simulink model "Code_2DoF_Simulation_Discrete"  (R2016b)
settings: Solver=FixedStepDiscrete  StartTime=0  StopTime=32  FixedStep=0.0025  MaxStep=0.005  MinStep=0.001  RelTol=0.5
undefined symbols (not defined in the file or in its folder): DiscIntNeverNeededParam
settings Model: ExtModeTrigMode=oneshot  ExtModeArmWhenConnect=off  Creator=hp  LastModifiedBy=sfijdl
settings DataIOCC: ExternalInput=untitled.getElement(1),[],[],[],[],[],[],[],[],[],[],[],[],[],[],[],[],[],[]  SaveFormat=Array  SignalLoggingSaveFormat=ModelDataLogs  SignalLoggingName=sigsOut
settings OptimizationCC: DefaultParameterBehavior=Inlined  UseDivisionForNetSlopeComputation=on  UseFloatMulNetSlope=on  InlineInvariantSignals=on  PassReuseOutputArgsAs=Individual arguments  ExpressionDepthLimit=2147483647  ZeroExternalMemoryAtStartup=off  ZeroInternalMemoryAtStartup=off  NoFixptDivByZeroProtection=on  EfficientFloat2IntCast=on  LifeSpan=1
settings DebuggingCC: SaveWithParameterizedLinksMsg=none  UnderspecifiedInitializationDetection=Classic  MergeDetectMultiDrivingBlocksExec=none  SignalResolutionControl=TryResolveAllWithWarning  MultiTaskDSMMsg=warning  MultiTaskCondExecSysMsg=none  MultiTaskRateTransMsg=warning  ParameterTunabilityLossMsg=error  FcnCallInpInsideContextMsg=warning  StateNameClashWarn=warning  SFUnexpectedBacktrackingDiag=warning  SFNoUnconditionalDefaultTransitionDiag=warning  SFExecutionAtInitializationDiag=none
settings HardwareCC: TargetBitPerPointer=64  TargetBitPerSizeT=64  TargetBitPerPtrDiffT=64  TargetLongLongMode=on  TargetIntDivRoundTo=Zero  TargetEndianess=LittleEndian  TargetWordSize=64  TargetHWDeviceType=MATLAB Host  ProdEqTarget=off
settings ModelReferenceCC: PropagateSignalLabelsOutOfModel=off
settings RTWCC: SystemTargetFile=ert.tlc  TemplateMakefile=ert_default_tmf  Description=Embedded Coder  GenerateReport=on  IncludeHyperlinkInReport=on  LaunchReport=on  GenerateTraceInfo=on  GenerateTraceReport=on  GenerateTraceReportSl=on  GenerateTraceReportSf=on  GenerateTraceReportEml=on  GenerateCodeMetricsReport=on
settings CodeAppCC: ForceParamTrailComments=on  IgnoreCustomStorageClasses=off  MaxIdLength=128  OperatorAnnotations=on  SimulinkDataObjDesc=on  SFDataObjDesc=on  MATLABFcnDesc=on  CustomSymbolStrGlobalVar=rt$N$M  CustomSymbolStrType=$N$M  CustomSymbolStrFcn=$N$M$F  CustomSymbolStrMacro=$N$M  InsertBlockDesc=on  MATLABSourceComments=on
settings ERTTargetCC: GenerateSampleERTMain=on  CombineSignalStateStructs=on  SupportComplex=off  SupportNonInlinedSFcns=on  InlinedParameterPlacement=NonHierarchical  ERTCustomFileTemplate=example_file_process.tlc  ERTFilePackagingFormat=CompactWithDataFile
settings ConfigComp: CovMetricSettings=dw  CovHtmlReporting=on  CovSaveCumulativeToWorkspaceVar=on  CovSaveSingleToWorkspaceVar=on  CovExternalEMLEnable=off

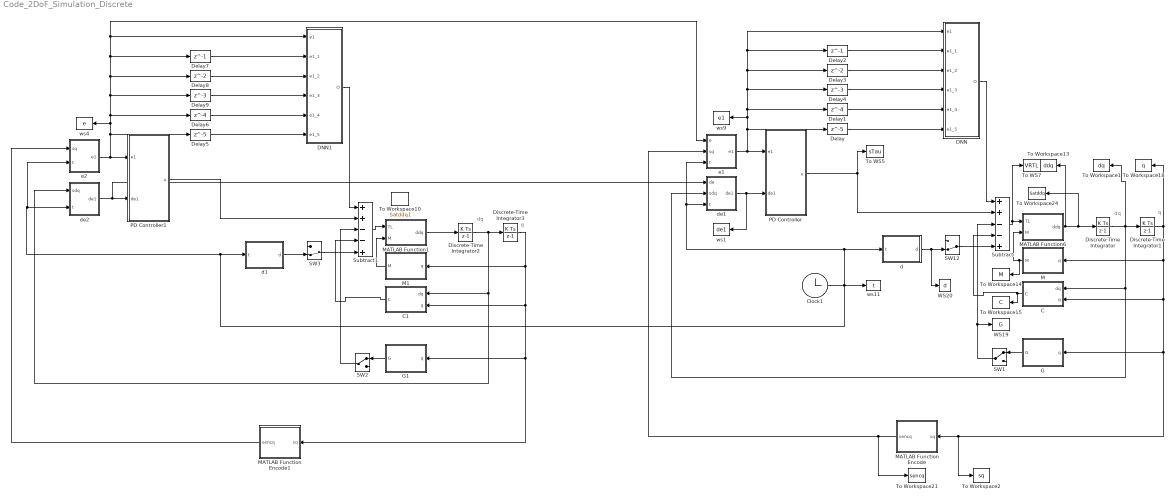
== system Code_2DoF_Simulation_Discrete ==
  note: q
  note: dq
  note: q
  note: dq
  C : MATLAB Function  TreatAsAtomicUnit=on
  C1 : MATLAB Function  TreatAsAtomicUnit=on
  Clock1 : Clock
  DNN : MATLAB Function  TreatAsAtomicUnit=on
  DNN1 : MATLAB Function  TreatAsAtomicUnit=on
  Delay : Delay  DelayLength=5  InitialCondition=0
  Delay1 : Delay  DelayLength=4  InitialCondition=0
  Delay2 : Delay  DelayLength=1  InitialCondition=0
  Delay3 : Delay  InitialCondition=0
  Delay4 : Delay  DelayLength=3  InitialCondition=0
  Delay5 : Delay  DelayLength=5  InitialCondition=0
  Delay6 : Delay  DelayLength=4  InitialCondition=0
  Delay7 : Delay  DelayLength=1  InitialCondition=0
  Delay8 : Delay  InitialCondition=0
  Delay9 : Delay  DelayLength=3  InitialCondition=0
  Discrete-Time Integrator : DiscreteIntegrator  InitialCondition=[0;0]  InitialConditionSetting=State (most efficient)  SampleTime=-1  ICPrevOutput=DiscIntNeverNeededParam  ICPrevScaledInput=DiscIntNeverNeededParam
  Discrete-Time Integrator1 : DiscreteIntegrator  InitialCondition=[-1;0]  InitialConditionSetting=State (most efficient)  SampleTime=-1  ICPrevOutput=DiscIntNeverNeededParam  ICPrevScaledInput=DiscIntNeverNeededParam
  Discrete-Time Integrator2 : DiscreteIntegrator  InitialCondition=[0;0]  InitialConditionSetting=State (most efficient)  SampleTime=-1  ICPrevOutput=DiscIntNeverNeededParam  ICPrevScaledInput=DiscIntNeverNeededParam
  Discrete-Time Integrator3 : DiscreteIntegrator  InitialCondition=[-1;0]  InitialConditionSetting=State (most efficient)  SampleTime=-1  ICPrevOutput=DiscIntNeverNeededParam  ICPrevScaledInput=DiscIntNeverNeededParam
  G : MATLAB Function  TreatAsAtomicUnit=on
  G1 : MATLAB Function  TreatAsAtomicUnit=on
  M : MATLAB Function  TreatAsAtomicUnit=on
  M1 : MATLAB Function  TreatAsAtomicUnit=on
  MATLAB Function Encode : MATLAB Function  TreatAsAtomicUnit=on
  MATLAB Function Encode1 : MATLAB Function  TreatAsAtomicUnit=on
  MATLAB Function1 : MATLAB Function  TreatAsAtomicUnit=on
  MATLAB Function6 : MATLAB Function  TreatAsAtomicUnit=on
  PD Controller : MATLAB Function  TreatAsAtomicUnit=on
  PD Controller1 : MATLAB Function  TreatAsAtomicUnit=on
  SW1 : ManualSwitch
  SW12 : ManualSwitch  CurrentSetting=0
  SW2 : ManualSwitch
  SW3 : ManualSwitch  CurrentSetting=0
  Subtract : Sum  Inputs=++--+
  Subtract1 : Sum  Inputs=++--+
  To WS5 : ToWorkspace  VariableName=sTau  SampleTime=-1
  To WS7 : ToWorkspace  VariableName=VRTL  SampleTime=-1
  To Workspace1 : ToWorkspace  VariableName=dq  SampleTime=-1
  To Workspace10 : ToWorkspace  VariableName=Satddq1  SampleTime=-1
  To Workspace13 : ToWorkspace  VariableName=ddq  SampleTime=-1
  To Workspace14 : ToWorkspace  VariableName=M  SampleTime=-1
  To Workspace15 : ToWorkspace  VariableName=C  SampleTime=-1
  To Workspace18 : ToWorkspace  VariableName=q  SampleTime=-1
  To Workspace2 : ToWorkspace  VariableName=sq  SampleTime=-1
  To Workspace21 : ToWorkspace  VariableName=sencq  SampleTime=-1
  To Workspace24 : ToWorkspace  VariableName=Satddq  SampleTime=-1
  WS19 : ToWorkspace  VariableName=G  SampleTime=-1
  WS20 : ToWorkspace  VariableName=d  SampleTime=-1
  d : MATLAB Function  TreatAsAtomicUnit=on
  d1 : MATLAB Function  TreatAsAtomicUnit=on
  de1 : MATLAB Function  TreatAsAtomicUnit=on
  de2 : MATLAB Function  TreatAsAtomicUnit=on
  e1 : MATLAB Function  TreatAsAtomicUnit=on
  e2 : MATLAB Function  TreatAsAtomicUnit=on
  ws1 : ToWorkspace  VariableName=de1  SampleTime=-1
  ws11 : ToWorkspace  VariableName=t  SampleTime=-1
  ws4 : ToWorkspace  VariableName=e  SampleTime=-1
  ws9 : ToWorkspace  VariableName=e1  SampleTime=-1
  wires:
  SW1/1 -> Subtract/3, WS19/1
  C/1(C) -> Subtract/4, To Workspace15/1
  Subtract/1 -> To WS7/1, MATLAB Function6/1(TL)
  M/1(M) -> MATLAB Function6/2(M), To Workspace14/1
  PD Controller/1(u) -> Subtract/2, To WS5/1
  Clock1/1 -> e2/2(t), de2/2(t), d1/1(t), ws11/1, e1/3(t), de1/3(t), d/1(t)
  Discrete-Time Integrator1/1 -> MATLAB Function Encode/1(sq), To Workspace2/1, G/1(q), C/2(q), M/1(q), To Workspace18/1
  MATLAB Function6/1(ddq) -> Discrete-Time Integrator/1, To Workspace24/1, To Workspace13/1
  de1/1(de1) -> ws1/1, PD Controller/2(de1)
  Discrete-Time Integrator/1 -> Discrete-Time Integrator1/1, To Workspace1/1, de1/2(sdq), C/1(dq)
  MATLAB Function Encode/1(sencq) -> To Workspace21/1, e1/2(sq)
  d/1(d) -> WS20/1, SW12/2
  SW12/1 -> Subtract/5
  G/1(G) -> SW1/1
  DNN/1(O) -> Subtract/1
  Delay/1 -> DNN/6(e1_5)
  Delay1/1 -> DNN/5(e1_4)
  Delay4/1 -> DNN/4(e1_3)
  Delay3/1 -> DNN/3(e1_2)
  Delay2/1 -> DNN/2(e1_1)
  e1/1(e1) -> PD Controller/1(e1), DNN/1(e1), Delay2/1, Delay3/1, Delay4/1, Delay1/1, ws9/1, Delay/1
  SW2/1 -> Subtract1/3
  C1/1(C) -> Subtract1/4
  Subtract1/1 -> MATLAB Function1/1(TL)
  M1/1(M) -> MATLAB Function1/2(M)
  PD Controller1/1(u) -> Subtract1/2
  Discrete-Time Integrator3/1 -> MATLAB Function Encode1/1(sq), G1/1(q), C1/2(q), M1/1(q)
  MATLAB Function1/1(ddq) -> Discrete-Time Integrator2/1
  de2/1(de1) -> de1/1(de), PD Controller1/2(de1)
  Discrete-Time Integrator2/1 -> Discrete-Time Integrator3/1, de2/1(sdq), C1/1(dq)
  MATLAB Function Encode1/1(sencq) -> e2/1(sq)
  d1/1(d) -> SW3/2
  SW3/1 -> Subtract1/5
  G1/1(G) -> SW2/1
  DNN1/1(O) -> Subtract1/1
  Delay5/1 -> DNN1/6(e1_5)
  Delay6/1 -> DNN1/5(e1_4)
  Delay9/1 -> DNN1/4(e1_3)
  Delay8/1 -> DNN1/3(e1_2)
  Delay7/1 -> DNN1/2(e1_1)
  e2/1(e1) -> PD Controller1/1(e1), e1/1(e), DNN1/1(e1), Delay7/1, Delay8/1, Delay9/1, Delay6/1, ws4/1, Delay5/1

== matlab function Code_2DoF_Simulation_Discrete/DNN ==
  settings: updateMethod=DISCRETE  sampleTime=0.0025
  data: e1 input; e1_1 input; e1_2 input; O output; e1_3 input; e1_4 input; e1_5 input
function O = DNN(e1,e1_1,e1_2,e1_3,e1_4,e1_5)
O=0;
end

== matlab function Code_2DoF_Simulation_Discrete/C1 ==
  settings: updateMethod=DISCRETE  sampleTime=0.0025
  data: dq input; C output; q input
function C = Col(dq,q)
q1=q(1);q2=q(2);
dq1=dq(1);dq2=dq(2);
s1=sin(q1);s2=sin(q2);
c1=cos(q1);c2=cos(q2);
m1=5;m2=5;
l1=1;l2=1;
g=9.81;
C11=-m2*l1*l2*s2*dq2;
C12=-m2*l1*l2*s2*dq2/2;
C21=m2*l1*l2*s2*dq1/2;
C22=0;
CM=[C11 C12
    C21 C22];
C=CM*dq;
end

== matlab function Code_2DoF_Simulation_Discrete/DNN1 ==
  settings: updateMethod=DISCRETE  sampleTime=0.0025
  data: e1 input; e1_1 input; e1_2 input; O output; e1_3 input; e1_4 input; e1_5 input
function O = DNN(e1,e1_1,e1_2,e1_3,e1_4,e1_5)
O=0;
end

== matlab function Code_2DoF_Simulation_Discrete/G1 ==
  settings: updateMethod=DISCRETE  sampleTime=0.0025
  data: q input; G output
function G = Gravity(q)
q1=q(1);q2=q(2);
s1=sin(q1);s2=sin(q2);
c1=cos(q1);c2=cos(q2);
c12=cos(q1+q2);
m1=5;m2=5;
l1=1;l2=1;
g=9.81;
G1 = m1*g*l1*c1/2+m2*g*l1*c1+m2*g*l2*c12/2; 
G2 = m2*g*l2*c12/2;
G=[G1;
   G2]; 
end

== matlab function Code_2DoF_Simulation_Discrete/M1 ==
  settings: updateMethod=DISCRETE  sampleTime=0.0025
  data: q input; M output
function M = Stiffness(q)
q1=q(1);q2=q(2);
s1=sin(q1);s2=sin(q2);
c1=cos(q1);c2=cos(q2);
m1=5;m2=5;
l1=1;l2=1;
g=9.81;
M11=m1*l1^2/3+m2*l1^2+m2*l2^2/4+m2*l1*l2*c2;
M12=m2*l2^2/4+m2*l1*l2*c2/2;
M22=m2*l2^2/3;
M = [M11; M12; 
     M12; M22];
end

== matlab function Code_2DoF_Simulation_Discrete/MATLAB Function Encode1 ==
  settings: updateMethod=DISCRETE  sampleTime=0.0025
  data: sq input; sencq output
function sencq = Enc(sq)
Delta=2*pi/2^19;
sencq=[0;0];
for i=1:1:2
    Number=floor(sq(i)/Delta)+1;
    sencq(i)=Number*Delta;
end
sencq=[sencq(1);sencq(2)];
% sencq=[sq(1);sq(2)];
end

== matlab function Code_2DoF_Simulation_Discrete/G ==
  settings: updateMethod=DISCRETE  sampleTime=0.0025
  data: q input; G output
function G = Gravity(q)
q1=q(1);q2=q(2);
s1=sin(q1);s2=sin(q2);
c1=cos(q1);c2=cos(q2);
c12=cos(q1+q2);
m1=5;m2=5;
l1=1;l2=1;
g=9.81;
G1 = m1*g*l1*c1/2+m2*g*l1*c1+m2*g*l2*c12/2; 
G2 = m2*g*l2*c12/2;
G=[G1;
   G2]; 
end

== matlab function Code_2DoF_Simulation_Discrete/MATLAB Function1 ==
  settings: updateMethod=DISCRETE  sampleTime=0.0025
  data: TL input; M input; ddq output
function ddq = Dynamics(TL,M)

M22 = [M(1) M(2)
       M(3) M(4)];
ddq=M22 \ TL;
end

== matlab function Code_2DoF_Simulation_Discrete/PD Controller1 ==
  settings: updateMethod=DISCRETE  sampleTime=0.0025
  data: e1 input; de1 input; u output
function u = Ctller(e1,de1)
% kp1=5000; kp2=1000; kd1=1000; kd2=80;
kp1=1000; kp2=800; kd1=500; kd2=80;
Kp=diag([kp1;kp2]);Kd=diag([kd1;kd2]);
u=-Kp*e1-Kd*de1;
end

== matlab function Code_2DoF_Simulation_Discrete/C ==
  settings: updateMethod=DISCRETE  sampleTime=0.0025
  data: dq input; C output; q input
function C = Col(dq,q)
q1=q(1);q2=q(2);
dq1=dq(1);dq2=dq(2);
s1=sin(q1);s2=sin(q2);
c1=cos(q1);c2=cos(q2);
m1=5;m2=5;
l1=1;l2=1;
g=9.81;
C11=-m2*l1*l2*s2*dq2;
C12=-m2*l1*l2*s2*dq2/2;
C21=m2*l1*l2*s2*dq1/2;
C22=0;
CM=[C11 C12
    C21 C22];
C=CM*dq;
end

== matlab function Code_2DoF_Simulation_Discrete/e1 ==
  settings: updateMethod=DISCRETE  sampleTime=0.0025
  data: e input; sq input; e1 output; t input
function e1 = e1(e,sq,t)
q=[sq(1);sq(2)];
qd1=sin(pi/4*t)-pi/2;
qd2=pi/2*cos(pi/8*(t+pi/2))*sin(pi/4*(t+pi/2));
% qd1=1;
% qd2=1;
qd=[qd1;qd2]; 
e1=q-qd;
e1=q-(qd-e1);
% e1=q-(qd-e);
end

== matlab function Code_2DoF_Simulation_Discrete/d1 ==
  settings: updateMethod=CONTINUOUS  sampleTime=0.0005
  data: t input; d output
function d = disturbance(t)
if t>10
% d=0.1*rand(6,1);
d=50.0*[sin(0.6*(t-10));sin(0.6*(t-10))];
else
    d=zeros(2,1);
% d=0.1*rand(6,1)*3*sin(0.5*t);
% d=0.3*sin(0.5*t)*ones(6,1);
end
end

== matlab function Code_2DoF_Simulation_Discrete/de2 ==
  settings: updateMethod=DISCRETE  sampleTime=0.0025
  data: sdq input; t input; de1 output
function de1 = de1(sdq,t)
dqd1=pi/4*cos(pi/4*t);
dqd2=pi/2*sin(pi/4*(t+pi/2))*-pi/8*sin(pi/8*(t+pi/2))+pi/2*cos(pi/8*(t+pi/2))*pi/4*cos(pi/4*(t+pi/2));
% dqd1=0;
% dqd2=0;
dqd=[dqd1;dqd2];
de1=sdq-dqd;
% de1=sdq-(dqd-de1);
end

== matlab function Code_2DoF_Simulation_Discrete/MATLAB Function6 ==
  settings: updateMethod=DISCRETE  sampleTime=0.0025
  data: TL input; M input; ddq output
function ddq = Dynamics(TL,M)

M22 = [M(1) M(2)
       M(3) M(4)];
ddq=M22 \ TL;
end

== matlab function Code_2DoF_Simulation_Discrete/e2 ==
  settings: updateMethod=DISCRETE  sampleTime=0.0025
  data: sq input; e1 output; t input
function e1 = e1(sq,t)
q=[sq(1);sq(2)];
qd1=sin(pi/4*t)-pi/2;
qd2=pi/2*cos(pi/8*(t+pi/2))*sin(pi/4*(t+pi/2));
% qd1=1;
% qd2=1;
qd=[qd1;qd2]; 
e1=q-qd;
% e1=q-(qd-e1);
end

== matlab function Code_2DoF_Simulation_Discrete/M ==
  settings: updateMethod=DISCRETE  sampleTime=0.0025
  data: q input; M output
function M = Stiffness(q)
q1=q(1);q2=q(2);
s1=sin(q1);s2=sin(q2);
c1=cos(q1);c2=cos(q2);
m1=5;m2=5;
l1=1;l2=1;
g=9.81;
M11=m1*l1^2/3+m2*l1^2+m2*l2^2/4+m2*l1*l2*c2;
M12=m2*l2^2/4+m2*l1*l2*c2/2;
M22=m2*l2^2/3;
M = [M11; M12; 
     M12; M22];
end

== matlab function Code_2DoF_Simulation_Discrete/d ==
  settings: updateMethod=CONTINUOUS  sampleTime=0.0005
  data: t input; d output
function d = disturbance(t)
if t>10
% d=0.1*rand(6,1);
d=50.0*[sin(0.6*(t-10));sin(0.6*(t-10))];
else
    d=zeros(2,1);
% d=0.1*rand(6,1)*3*sin(0.5*t);
% d=0.3*sin(0.5*t)*ones(6,1);
end
end

== matlab function Code_2DoF_Simulation_Discrete/MATLAB Function Encode ==
  settings: updateMethod=DISCRETE  sampleTime=0.0025
  data: sq input; sencq output
function sencq = Enc(sq)
Delta=2*pi/2^19;
sencq=[0;0];
for i=1:1:2
    Number=floor(sq(i)/Delta)+1;
    sencq(i)=Number*Delta;
end
sencq=[sencq(1);sencq(2)];
% sencq=[sq(1);sq(2)];
end

== matlab function Code_2DoF_Simulation_Discrete/PD Controller ==
  settings: updateMethod=DISCRETE  sampleTime=0.0025
  data: e1 input; de1 input; u output
function u = Ctller(e1,de1)
% kp1=5000; kp2=1000; kd1=1000; kd2=80;
kp1=1000; kp2=800; kd1=500; kd2=80;
Kp=diag([kp1;kp2]);Kd=diag([kd1;kd2]);
u=-Kp*e1-Kd*de1;
end

== matlab function Code_2DoF_Simulation_Discrete/de1 ==
  settings: updateMethod=DISCRETE  sampleTime=0.0025
  data: de input; sdq input; t input; de1 output
function de1 = de1(de,sdq,t)
dqd1=pi/4*cos(pi/4*t);
dqd2=pi/2*sin(pi/4*(t+pi/2))*-pi/8*sin(pi/8*(t+pi/2))+pi/2*cos(pi/8*(t+pi/2))*pi/4*cos(pi/4*(t+pi/2));
% dqd1=0;
% dqd2=0;
dqd=[dqd1;dqd2];
de1=sdq-dqd;
de1=sdq-(dqd-de1);
% de1=sdq-(dqd-de);
end
